simulink model "pedal_project"  (R2025b)
settings: Solver=VariableStepAuto  StartTime=0.0  StopTime=10.0  RelTol=1e-3
(part 1 of 2)

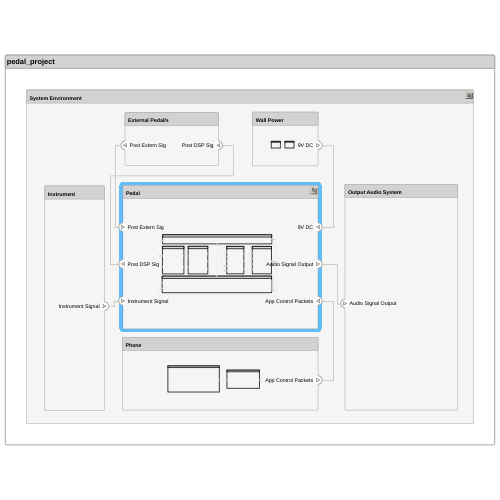
[thumbnail: Simulink's stored preview of the top-level diagram]
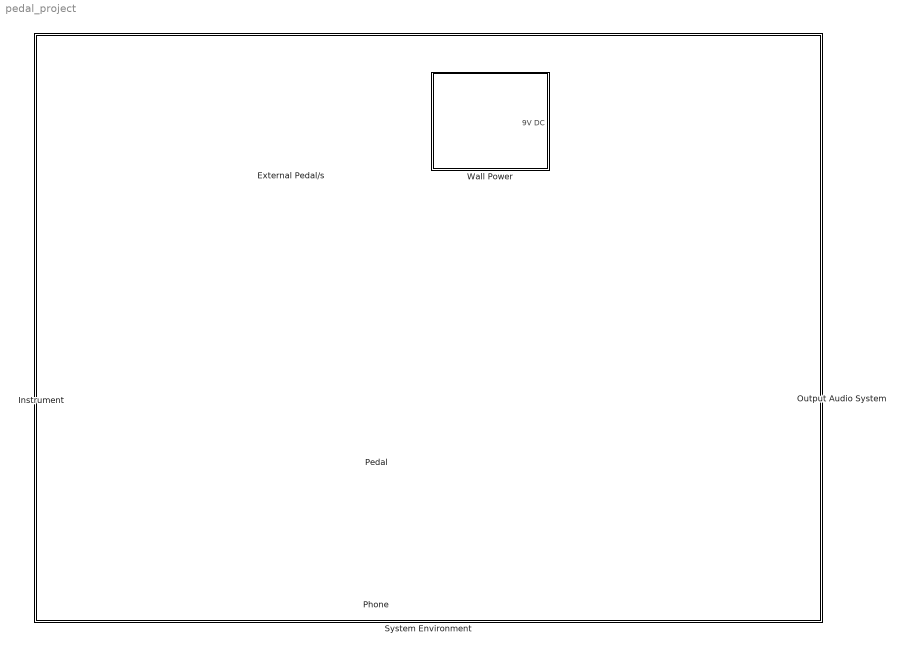
== system pedal_project ==
  External Pedal/s : Subsystem
      settings: PortSchema="{\"entries\":[{\"content\":{\"headerSize\":26,\"margin\":15,\"minimumSpacing\":25,\"sides\":[{\"content\":{\"connectorIds\":[\"Out1\"]},\"type\":\"ConnectorPlacement.EquallySpacedRectSide\",\"uuid\":\"d45e420a-c48a-4f64-96ce-c5c35bb4ca1a\"},{\"content\":{\"connectorIds\":[\"In1\"],\"side\":\"RIGHT\"},\"type\":\"ConnectorPlacement.EquallySpacedRectSide\",\"uuid\":\"a4e2bce0-d957-4e8d-907b-26e945724fec\"},{\"content\":{\"side\":\"TOP\"},\"type\":\"ConnectorPlacement.EquallySpacedRectSide\",\"uuid\":\"f887741f-84ea-4dc9-b916-61633ba77119\"},{\"content\":{\"side\":\"BOTTOM\"},\"type\":\"ConnectorPlacement.EquallySpacedRectSide\",\"uuid\":\"3b146cbf-c6c6-4afe-90ef-4dca6329af2e\"}]},\"type\":\"ConnectorPlacement.EquallySpacedConnector\",\"uuid\":\"ffda6ec7-3a8c-4734-85c7-d4d2baf408ab\"}],\"packageUris\":[\"http://schema.mathworks.com/mf0/Connector/R2020b\"],\"version\":\"1.0\"}"
  Instrument : Subsystem
      settings: PortSchema="{\"entries\":[{\"content\":{\"headerSize\":26,\"margin\":15,\"minimumSpacing\":25,\"sides\":[{\"content\":{},\"type\":\"ConnectorPlacement.EquallySpacedRectSide\",\"uuid\":\"d45e420a-c48a-4f64-96ce-c5c35bb4ca1a\"},{\"content\":{\"connectorIds\":[\"Out1\"],\"side\":\"RIGHT\"},\"type\":\"ConnectorPlacement.EquallySpacedRectSide\",\"uuid\":\"a4e2bce0-d957-4e8d-907b-26e945724fec\"},{\"content\":{\"side\":\"TOP\"},\"type\":\"ConnectorPlacement.EquallySpacedRectSide\",\"uuid\":\"f887741f-84ea-4dc9-b916-61633ba77119\"}]},\"type\":\"ConnectorPlacement.EquallySpacedConnector\",\"uuid\":\"ffda6ec7-3a8c-4734-85c7-d4d2baf408ab\"}],\"packageUris\":[\"http://schema.mathworks.com/mf0/Connector/R2020b\"],\"version\":\"1.0\"}"
  Output Audio System : Subsystem
      settings: PortSchema="{\"entries\":[{\"content\":{\"headerSize\":26,\"margin\":15,\"minimumSpacing\":25,\"sides\":[{\"content\":{\"connectorIds\":[\"In1\"]},\"type\":\"ConnectorPlacement.EquallySpacedRectSide\",\"uuid\":\"d45e420a-c48a-4f64-96ce-c5c35bb4ca1a\"},{\"content\":{\"side\":\"RIGHT\"},\"type\":\"ConnectorPlacement.EquallySpacedRectSide\",\"uuid\":\"a4e2bce0-d957-4e8d-907b-26e945724fec\"},{\"content\":{\"side\":\"TOP\"},\"type\":\"ConnectorPlacement.EquallySpacedRectSide\",\"uuid\":\"f887741f-84ea-4dc9-b916-61633ba77119\"}]},\"type\":\"ConnectorPlacement.EquallySpacedConnector\",\"uuid\":\"ffda6ec7-3a8c-4734-85c7-d4d2baf408ab\"}],\"packageUris\":[\"http://schema.mathworks.com/mf0/Connector/R2020b\"],\"version\":\"1.0\"}"
  Pedal : Subsystem
      settings: PortSchema="{\"entries\":[{\"content\":{\"headerSize\":26,\"margin\":15,\"minimumSpacing\":25,\"sides\":[{\"content\":{\"connectorIds\":[\"In3\",\"Out2\",\"In4\"]},\"type\":\"ConnectorPlacement.EquallySpacedRectSide\",\"uuid\":\"d45e420a-c48a-4f64-96ce-c5c35bb4ca1a\"},{\"content\":{\"connectorIds\":[\"In1\",\"Out1\",\"In2\"],\"side\":\"RIGHT\"},\"type\":\"ConnectorPlacement.EquallySpacedRectSide\",\"uuid\":\"a4e2bce0-d957-4e8d-907b-26e945724fec\"},{\"content\":{\"side\":\"TOP\"},\"type\":\"ConnectorPlacement.EquallySpacedRectSide\",\"uuid\":\"f887741f-84ea-4dc9-b916-61633ba77119\"}]},\"type\":\"ConnectorPlacement.EquallySpacedConnector\",\"uuid\":\"ffda6ec7-3a8c-4734-85c7-d4d2baf408ab\"}],\"packageUris\":[\"http://schema.mathworks.com/mf0/Connector/R2020b\"],\"version\":\"1.0\"}"
  Phone : Subsystem
      settings: PortSchema="{\"entries\":[{\"content\":{\"headerSize\":26,\"margin\":15,\"minimumSpacing\":25,\"sides\":[{\"content\":{},\"type\":\"ConnectorPlacement.EquallySpacedRectSide\",\"uuid\":\"d45e420a-c48a-4f64-96ce-c5c35bb4ca1a\"},{\"content\":{\"connectorIds\":[\"Out1\"],\"side\":\"RIGHT\"},\"type\":\"ConnectorPlacement.EquallySpacedRectSide\",\"uuid\":\"a4e2bce0-d957-4e8d-907b-26e945724fec\"},{\"content\":{\"side\":\"TOP\"},\"type\":\"ConnectorPlacement.EquallySpacedRectSide\",\"uuid\":\"f887741f-84ea-4dc9-b916-61633ba77119\"}]},\"type\":\"ConnectorPlacement.EquallySpacedConnector\",\"uuid\":\"ffda6ec7-3a8c-4734-85c7-d4d2baf408ab\"}],\"packageUris\":[\"http://schema.mathworks.com/mf0/Connector/R2020b\"],\"version\":\"1.0\"}"
  System Environment : Subsystem
      settings: PortSchema="{\"entries\":[{\"content\":{\"headerSize\":26,\"margin\":15,\"minimumSpacing\":25,\"sides\":[{\"content\":{},\"type\":\"ConnectorPlacement.EquallySpacedRectSide\",\"uuid\":\"ff6d08b7-25e5-4e55-8f49-6be1cf87a249\"},{\"content\":{\"side\":\"RIGHT\"},\"type\":\"ConnectorPlacement.EquallySpacedRectSide\",\"uuid\":\"cf714437-3edf-4193-96f0-527040f4845b\"},{\"content\":{\"side\":\"TOP\"},\"type\":\"ConnectorPlacement.EquallySpacedRectSide\",\"uuid\":\"edc7f9df-45d2-49f5-b248-99123dbc3df5\"}]},\"type\":\"ConnectorPlacement.EquallySpacedConnector\",\"uuid\":\"82090768-c12d-4d7c-bb71-6334bd2f3885\"}],\"packageUris\":[\"http://schema.mathworks.com/mf0/Connector/R2020b\"],\"version\":\"1.0\"}"
  Wall Power : Subsystem
      settings: PortSchema="{\"entries\":[{\"content\":{\"headerSize\":26,\"margin\":15,\"minimumSpacing\":25,\"sides\":[{\"content\":{},\"type\":\"ConnectorPlacement.EquallySpacedRectSide\",\"uuid\":\"d45e420a-c48a-4f64-96ce-c5c35bb4ca1a\"},{\"content\":{\"connectorIds\":[\"Out1\"],\"side\":\"RIGHT\"},\"type\":\"ConnectorPlacement.EquallySpacedRectSide\",\"uuid\":\"a4e2bce0-d957-4e8d-907b-26e945724fec\"},{\"content\":{\"side\":\"TOP\"},\"type\":\"ConnectorPlacement.EquallySpacedRectSide\",\"uuid\":\"f887741f-84ea-4dc9-b916-61633ba77119\"},{\"content\":{\"side\":\"BOTTOM\"},\"type\":\"ConnectorPlacement.EquallySpacedRectSide\",\"uuid\":\"d7988f96-c3a6-4963-bdc5-536baf489e90\"}]},\"type\":\"ConnectorPlacement.EquallySpacedConnector\",\"uuid\":\"ffda6ec7-3a8c-4734-85c7-d4d2baf408ab\"}],\"packageUris\":[\"http://schema.mathworks.com/mf0/Connector/R2020b\"],\"version\":\"1.0\"}"
  wires:
  Instrument/1(Instrument Signal) -> Pedal/4(Instrument Signal)
  Pedal/2(Post DSP Sig) -> External Pedal/s/1(Post DSP Sig)
  External Pedal/s/1(Post Extern Sig) -> Pedal/3(Post Extern Sig)
  Wall Power/1(9V DC) -> Pedal/1(9V DC)
  Phone/1(App Control Packets) -> Pedal/2(App Control Packets)
  Pedal/1(Audio Signal Output) -> Output Audio System/1(Audio Signal Output)

== system pedal_project/External Pedal//s ==
  Bus Element In1 : Inport  PortName=Post DSP Sig
  Bus Element Out1 : Outport  PortName=Post Extern Sig

== system pedal_project/Instrument ==
  Bus Element Out1 : Outport  PortName=Instrument Signal

== system pedal_project/Output Audio System ==
  Bus Element In1 : Inport  PortName=Audio Signal Output

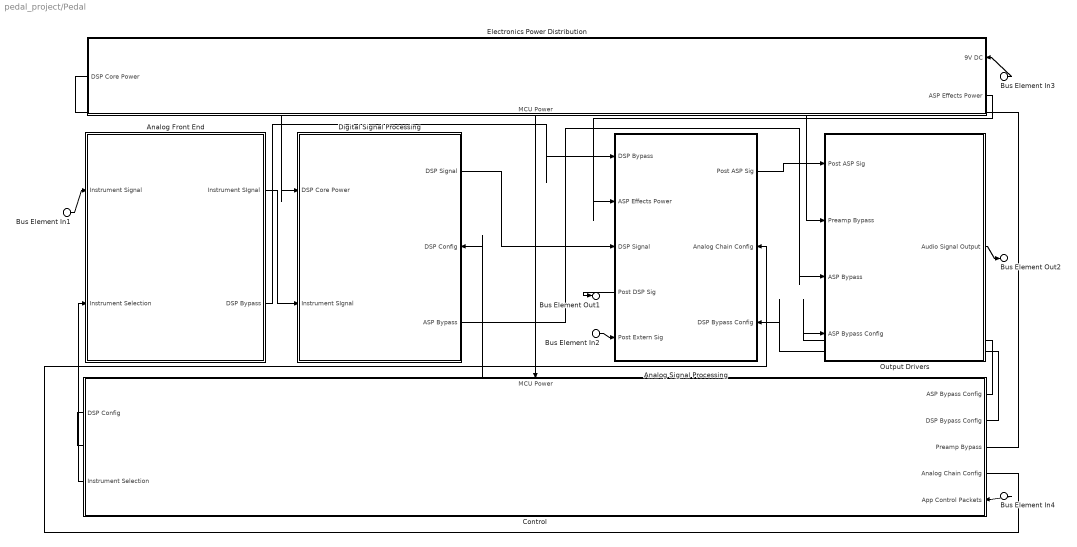
== system pedal_project/Pedal ==
  Bus Element In3 : Inport  PortName=9V DC
  Bus Element In4 : Inport  Port=2  PortName=App Control Packets
  Bus Element In2 : Inport  Port=3  PortName=Post Extern Sig
  Bus Element In1 : Inport  Port=4  PortName=Instrument Signal
  Analog Front End : Subsystem
      settings: PortSchema="{\"entries\":[{\"content\":{\"headerSize\":26,\"margin\":15,\"minimumSpacing\":25,\"sides\":[{\"content\":{\"connectorIds\":[\"In1\",\"In2\"]},\"type\":\"ConnectorPlacement.EquallySpacedRectSide\",\"uuid\":\"d45e420a-c48a-4f64-96ce-c5c35bb4ca1a\"},{\"content\":{\"connectorIds\":[\"Out1\",\"Out2\"],\"side\":\"RIGHT\"},\"type\":\"ConnectorPlacement.EquallySpacedRectSide\",\"uuid\":\"a4e2bce0-d957-4e8d-907b-26e945724fec\"},{\"content\":{\"side\":\"TOP\"},\"type\":\"ConnectorPlacement.EquallySpacedRectSide\",\"uuid\":\"f887741f-84ea-4dc9-b916-61633ba77119\"}]},\"type\":\"ConnectorPlacement.EquallySpacedConnector\",\"uuid\":\"ffda6ec7-3a8c-4734-85c7-d4d2baf408ab\"}],\"packageUris\":[\"http://schema.mathworks.com/mf0/Connector/R2020b\"],\"version\":\"1.0\"}"
  Analog Signal Processing : Subsystem
      settings: PortSchema="{\"entries\":[{\"content\":{\"headerSize\":26,\"margin\":15,\"minimumSpacing\":25,\"sides\":[{\"content\":{\"connectorIds\":[\"In1\",\"In3\",\"In4\",\"Out1\",\"In6\"]},\"type\":\"ConnectorPlacement.EquallySpacedRectSide\",\"uuid\":\"d45e420a-c48a-4f64-96ce-c5c35bb4ca1a\"},{\"content\":{\"connectorIds\":[\"Out2\",\"In5\",\"In2\"],\"side\":\"RIGHT\"},\"type\":\"ConnectorPlacement.EquallySpacedRectSide\",\"uuid\":\"a4e2bce0-d957-4e8d-907b-26e945724fec\"},{\"content\":{\"side\":\"TOP\"},\"type\":\"ConnectorPlacement.EquallySpacedRectSide\",\"uuid\":\"f887741f-84ea-4dc9-b916-61633ba77119\"}]},\"type\":\"ConnectorPlacement.EquallySpacedConnector\",\"uuid\":\"ffda6ec7-3a8c-4734-85c7-d4d2baf408ab\"}],\"packageUris\":[\"http://schema.mathworks.com/mf0/Connector/R2020b\"],\"version\":\"1.0\"}"
  Control : Subsystem
      settings: PortSchema="{\"entries\":[{\"content\":{\"headerSize\":26,\"margin\":15,\"minimumSpacing\":25,\"sides\":[{\"content\":{\"connectorIds\":[\"Out4\",\"Out5\"]},\"type\":\"ConnectorPlacement.EquallySpacedRectSide\",\"uuid\":\"d45e420a-c48a-4f64-96ce-c5c35bb4ca1a\"},{\"content\":{\"connectorIds\":[\"Out1\",\"Out2\",\"Out3\",\"Out6\",\"In1\"],\"side\":\"RIGHT\"},\"type\":\"ConnectorPlacement.EquallySpacedRectSide\",\"uuid\":\"a4e2bce0-d957-4e8d-907b-26e945724fec\"},{\"content\":{\"connectorIds\":[\"In2\"],\"side\":\"TOP\"},\"type\":\"ConnectorPlacement.EquallySpacedRectSide\",\"uuid\":\"f887741f-84ea-4dc9-b916-61633ba77119\"}]},\"type\":\"ConnectorPlacement.EquallySpacedConnector\",\"uuid\":\"ffda6ec7-3a8c-4734-85c7-d4d2baf408ab\"}],\"packageUris\":[\"http://schema.mathworks.com/mf0/Connector/R2020b\"],\"version\":\"1.0\"}"
  Digital Signal Processing : Subsystem
      settings: PortSchema="{\"entries\":[{\"content\":{\"headerSize\":26,\"margin\":15,\"minimumSpacing\":25,\"sides\":[{\"content\":{\"connectorIds\":[\"In1\",\"In3\"]},\"type\":\"ConnectorPlacement.EquallySpacedRectSide\",\"uuid\":\"d45e420a-c48a-4f64-96ce-c5c35bb4ca1a\"},{\"content\":{\"connectorIds\":[\"Out1\",\"In2\",\"Out2\"],\"side\":\"RIGHT\"},\"type\":\"ConnectorPlacement.EquallySpacedRectSide\",\"uuid\":\"a4e2bce0-d957-4e8d-907b-26e945724fec\"},{\"content\":{\"side\":\"TOP\"},\"type\":\"ConnectorPlacement.EquallySpacedRectSide\",\"uuid\":\"f887741f-84ea-4dc9-b916-61633ba77119\"}]},\"type\":\"ConnectorPlacement.EquallySpacedConnector\",\"uuid\":\"ffda6ec7-3a8c-4734-85c7-d4d2baf408ab\"}],\"packageUris\":[\"http://schema.mathworks.com/mf0/Connector/R2020b\"],\"version\":\"1.0\"}"
  Electronics Power Distribution : Subsystem
      settings: PortSchema="{\"entries\":[{\"content\":{\"headerSize\":26,\"margin\":15,\"minimumSpacing\":25,\"sides\":[{\"content\":{\"connectorIds\":[\"Out2\"]},\"type\":\"ConnectorPlacement.EquallySpacedRectSide\",\"uuid\":\"d45e420a-c48a-4f64-96ce-c5c35bb4ca1a\"},{\"content\":{\"connectorIds\":[\"In1\",\"Out1\"],\"side\":\"RIGHT\"},\"type\":\"ConnectorPlacement.EquallySpacedRectSide\",\"uuid\":\"a4e2bce0-d957-4e8d-907b-26e945724fec\"},{\"content\":{\"side\":\"TOP\"},\"type\":\"ConnectorPlacement.EquallySpacedRectSide\",\"uuid\":\"f887741f-84ea-4dc9-b916-61633ba77119\"},{\"content\":{\"connectorIds\":[\"Out3\"],\"side\":\"BOTTOM\"},\"type\":\"ConnectorPlacement.EquallySpacedRectSide\",\"uuid\":\"c9173022-6e53-493b-a07b-56b093cd8358\"}]},\"type\":\"ConnectorPlacement.EquallySpacedConnector\",\"uuid\":\"ffda6ec7-3a8c-4734-85c7-d4d2baf408ab\"}],\"packageUris\":[\"http://schema.mathworks.com/mf0/Connector/R2020b\"],\"version\":\"1.0\"}"
  Output Drivers : Subsystem
      settings: PortSchema="{\"entries\":[{\"content\":{\"headerSize\":26,\"margin\":15,\"minimumSpacing\":25,\"sides\":[{\"content\":{\"connectorIds\":[\"In1\",\"In2\",\"In3\",\"In4\"]},\"type\":\"ConnectorPlacement.EquallySpacedRectSide\",\"uuid\":\"d45e420a-c48a-4f64-96ce-c5c35bb4ca1a\"},{\"content\":{\"connectorIds\":[\"Out1\"],\"side\":\"RIGHT\"},\"type\":\"ConnectorPlacement.EquallySpacedRectSide\",\"uuid\":\"a4e2bce0-d957-4e8d-907b-26e945724fec\"},{\"content\":{\"side\":\"TOP\"},\"type\":\"ConnectorPlacement.EquallySpacedRectSide\",\"uuid\":\"f887741f-84ea-4dc9-b916-61633ba77119\"}]},\"type\":\"ConnectorPlacement.EquallySpacedConnector\",\"uuid\":\"ffda6ec7-3a8c-4734-85c7-d4d2baf408ab\"}],\"packageUris\":[\"http://schema.mathworks.com/mf0/Connector/R2020b\"],\"version\":\"1.0\"}"
  Bus Element Out2 : Outport  PortName=Audio Signal Output
  Bus Element Out1 : Outport  Port=2  PortName=Post DSP Sig
  wires:
  Electronics Power Distribution/3(MCU Power) -> Control/2(MCU Power)
  Bus Element In4/1 -> Control/1(App Control Packets)
  Output Drivers/1(Audio Signal Output) -> Bus Element Out2/1
  Bus Element In3/1 -> Electronics Power Distribution/1(9V DC)
  Bus Element In2/1 -> Analog Signal Processing/6(Post Extern Sig)
  Bus Element In1/1 -> Analog Front End/1(Instrument Signal)
  Analog Front End/1(Instrument SIgnal) -> Digital Signal Processing/3(Instrument SIgnal)
  Analog Signal Processing/2(Post ASP Sig) -> Output Drivers/1(Post ASP Sig)
  Control/6(Analog Chain Config) -> Analog Signal Processing/5(Analog Chain Config)
  Control/4(DSP Config) -> Digital Signal Processing/2(DSP Config)
  Control/5(Instrument Selection) -> Analog Front End/2(Instrument Selection)
  Electronics Power Distribution/2(DSP Core Power) -> Digital Signal Processing/1(DSP Core Power)
  Electronics Power Distribution/1(ASP Effects Power) -> Analog Signal Processing/3(ASP Effects Power)
  Analog Signal Processing/1(Post DSP Sig) -> Bus Element Out1/1
  Digital Signal Processing/1(DSP Signal) -> Analog Signal Processing/4(DSP Signal)
  Control/3(Preamp Bypass) -> Output Drivers/2(Preamp Bypass)
  Digital Signal Processing/2(ASP Bypass) -> Output Drivers/3(ASP Bypass)
  Analog Front End/2(DSP Bypass) -> Analog Signal Processing/1(DSP Bypass)
  Control/2(DSP Bypass Config) -> Analog Signal Processing/2(DSP Bypass Config)
  Control/1(ASP Bypass Config) -> Output Drivers/4(ASP Bypass Config)

== system pedal_project/Phone ==
  Software Application : Subsystem
      settings: PortSchema="{\"entries\":[{\"content\":{\"headerSize\":26,\"margin\":15,\"minimumSpacing\":25,\"sides\":[{\"content\":{},\"type\":\"ConnectorPlacement.EquallySpacedRectSide\",\"uuid\":\"d45e420a-c48a-4f64-96ce-c5c35bb4ca1a\"},{\"content\":{\"connectorIds\":[\"Out1\"],\"side\":\"RIGHT\"},\"type\":\"ConnectorPlacement.EquallySpacedRectSide\",\"uuid\":\"a4e2bce0-d957-4e8d-907b-26e945724fec\"},{\"content\":{\"side\":\"TOP\"},\"type\":\"ConnectorPlacement.EquallySpacedRectSide\",\"uuid\":\"f887741f-84ea-4dc9-b916-61633ba77119\"}]},\"type\":\"ConnectorPlacement.EquallySpacedConnector\",\"uuid\":\"ffda6ec7-3a8c-4734-85c7-d4d2baf408ab\"}],\"packageUris\":[\"http://schema.mathworks.com/mf0/Connector/R2020b\"],\"version\":\"1.0\"}"
  USB Output Driver : Subsystem
      settings: PortSchema="{\"entries\":[{\"content\":{\"headerSize\":26,\"margin\":15,\"minimumSpacing\":25,\"sides\":[{\"content\":{\"connectorIds\":[\"In1\"]},\"type\":\"ConnectorPlacement.EquallySpacedRectSide\",\"uuid\":\"d45e420a-c48a-4f64-96ce-c5c35bb4ca1a\"},{\"content\":{\"connectorIds\":[\"Out1\"],\"side\":\"RIGHT\"},\"type\":\"ConnectorPlacement.EquallySpacedRectSide\",\"uuid\":\"a4e2bce0-d957-4e8d-907b-26e945724fec\"},{\"content\":{\"side\":\"TOP\"},\"type\":\"ConnectorPlacement.EquallySpacedRectSide\",\"uuid\":\"f887741f-84ea-4dc9-b916-61633ba77119\"}]},\"type\":\"ConnectorPlacement.EquallySpacedConnector\",\"uuid\":\"ffda6ec7-3a8c-4734-85c7-d4d2baf408ab\"}],\"packageUris\":[\"http://schema.mathworks.com/mf0/Connector/R2020b\"],\"version\":\"1.0\"}"
  Bus Element Out1 : Outport  PortName=App Control Packets
  wires:
  USB Output Driver/1(App Control Packets) -> Bus Element Out1/1
  Software Application/1(Configuration Upload Packets) -> USB Output Driver/1(Configuration Upload Packets)

== system pedal_project/System Environment ==

== system pedal_project/Wall Power ==
  120V Wall Output : Subsystem
      settings: PortSchema="{\"entries\":[{\"content\":{\"headerSize\":26,\"margin\":15,\"minimumSpacing\":25,\"sides\":[{\"content\":{},\"type\":\"ConnectorPlacement.EquallySpacedRectSide\",\"uuid\":\"d45e420a-c48a-4f64-96ce-c5c35bb4ca1a\"},{\"content\":{\"connectorIds\":[\"Out1\"],\"side\":\"RIGHT\"},\"type\":\"ConnectorPlacement.EquallySpacedRectSide\",\"uuid\":\"a4e2bce0-d957-4e8d-907b-26e945724fec\"},{\"content\":{\"side\":\"TOP\"},\"type\":\"ConnectorPlacement.EquallySpacedRectSide\",\"uuid\":\"f887741f-84ea-4dc9-b916-61633ba77119\"}]},\"type\":\"ConnectorPlacement.EquallySpacedConnector\",\"uuid\":\"ffda6ec7-3a8c-4734-85c7-d4d2baf408ab\"}],\"packageUris\":[\"http://schema.mathworks.com/mf0/Connector/R2020b\"],\"version\":\"1.0\"}"
  9V DC Power Supply : Subsystem
      settings: PortSchema="{\"entries\":[{\"content\":{\"headerSize\":26,\"margin\":15,\"minimumSpacing\":25,\"sides\":[{\"content\":{\"connectorIds\":[\"In1\"]},\"type\":\"ConnectorPlacement.EquallySpacedRectSide\",\"uuid\":\"d45e420a-c48a-4f64-96ce-c5c35bb4ca1a\"},{\"content\":{\"connectorIds\":[\"Out1\"],\"side\":\"RIGHT\"},\"type\":\"ConnectorPlacement.EquallySpacedRectSide\",\"uuid\":\"a4e2bce0-d957-4e8d-907b-26e945724fec\"},{\"content\":{\"side\":\"TOP\"},\"type\":\"ConnectorPlacement.EquallySpacedRectSide\",\"uuid\":\"f887741f-84ea-4dc9-b916-61633ba77119\"}]},\"type\":\"ConnectorPlacement.EquallySpacedConnector\",\"uuid\":\"ffda6ec7-3a8c-4734-85c7-d4d2baf408ab\"}],\"packageUris\":[\"http://schema.mathworks.com/mf0/Connector/R2020b\"],\"version\":\"1.0\"}"
  Bus Element Out1 : Outport  PortName=9V DC
  wires:
  120V Wall Output/1(Wall Power) -> 9V DC Power Supply/1(Wall Power)
  9V DC Power Supply/1(9V DC) -> Bus Element Out1/1

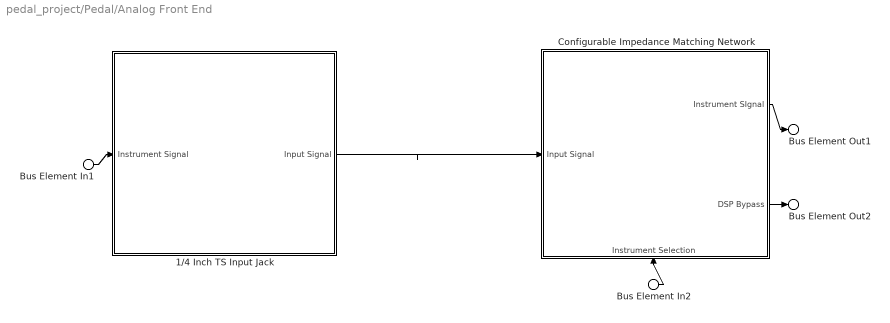
== system pedal_project/Pedal/Analog Front End ==
  Bus Element In1 : Inport  PortName=Instrument Signal
  Bus Element In2 : Inport  Port=2  PortName=Instrument Selection
  1/4 Inch TS Input Jack : Subsystem
      settings: PortSchema="{\"entries\":[{\"content\":{\"headerSize\":26,\"margin\":15,\"minimumSpacing\":25,\"sides\":[{\"content\":{\"connectorIds\":[\"In1\"]},\"type\":\"ConnectorPlacement.EquallySpacedRectSide\",\"uuid\":\"d45e420a-c48a-4f64-96ce-c5c35bb4ca1a\"},{\"content\":{\"connectorIds\":[\"Out1\"],\"side\":\"RIGHT\"},\"type\":\"ConnectorPlacement.EquallySpacedRectSide\",\"uuid\":\"a4e2bce0-d957-4e8d-907b-26e945724fec\"},{\"content\":{\"side\":\"TOP\"},\"type\":\"ConnectorPlacement.EquallySpacedRectSide\",\"uuid\":\"f887741f-84ea-4dc9-b916-61633ba77119\"}]},\"type\":\"ConnectorPlacement.EquallySpacedConnector\",\"uuid\":\"ffda6ec7-3a8c-4734-85c7-d4d2baf408ab\"}],\"packageUris\":[\"http://schema.mathworks.com/mf0/Connector/R2020b\"],\"version\":\"1.0\"}"
  Configurable Impedance Matching Network : Subsystem
      settings: PortSchema="{\"entries\":[{\"content\":{\"headerSize\":26,\"margin\":15,\"minimumSpacing\":25,\"sides\":[{\"content\":{\"connectorIds\":[\"In2\"]},\"type\":\"ConnectorPlacement.EquallySpacedRectSide\",\"uuid\":\"d45e420a-c48a-4f64-96ce-c5c35bb4ca1a\"},{\"content\":{\"connectorIds\":[\"Out1\",\"Out2\"],\"side\":\"RIGHT\"},\"type\":\"ConnectorPlacement.EquallySpacedRectSide\",\"uuid\":\"a4e2bce0-d957-4e8d-907b-26e945724fec\"},{\"content\":{\"side\":\"TOP\"},\"type\":\"ConnectorPlacement.EquallySpacedRectSide\",\"uuid\":\"f887741f-84ea-4dc9-b916-61633ba77119\"},{\"content\":{\"connectorIds\":[\"In1\"],\"side\":\"BOTTOM\"},\"type\":\"ConnectorPlacement.EquallySpacedRectSide\",\"uuid\":\"a508731f-4cdb-4416-a773-6d2230bc93f7\"}]},\"type\":\"ConnectorPlacement.EquallySpacedConnector\",\"uuid\":\"ffda6ec7-3a8c-4734-85c7-d4d2baf408ab\"}],\"packageUris\":[\"http://schema.mathworks.com/mf0/Connector/R2020b\"],\"version\":\"1.0\"}"
  Bus Element Out1 : Outport  PortName=Instrument SIgnal
  Bus Element Out2 : Outport  Port=2  PortName=DSP Bypass
  wires:
  Bus Element In1/1 -> 1/4 Inch TS Input Jack/1(Instrument Signal)
  1/4 Inch TS Input Jack/1(Input Signal) -> Configurable Impedance Matching Network/2(Input Signal)
  Configurable Impedance Matching Network/1(Instrument SIgnal) -> Bus Element Out1/1
  Bus Element In2/1 -> Configurable Impedance Matching Network/1(Instrument Selection)
  Configurable Impedance Matching Network/2(DSP Bypass) -> Bus Element Out2/1

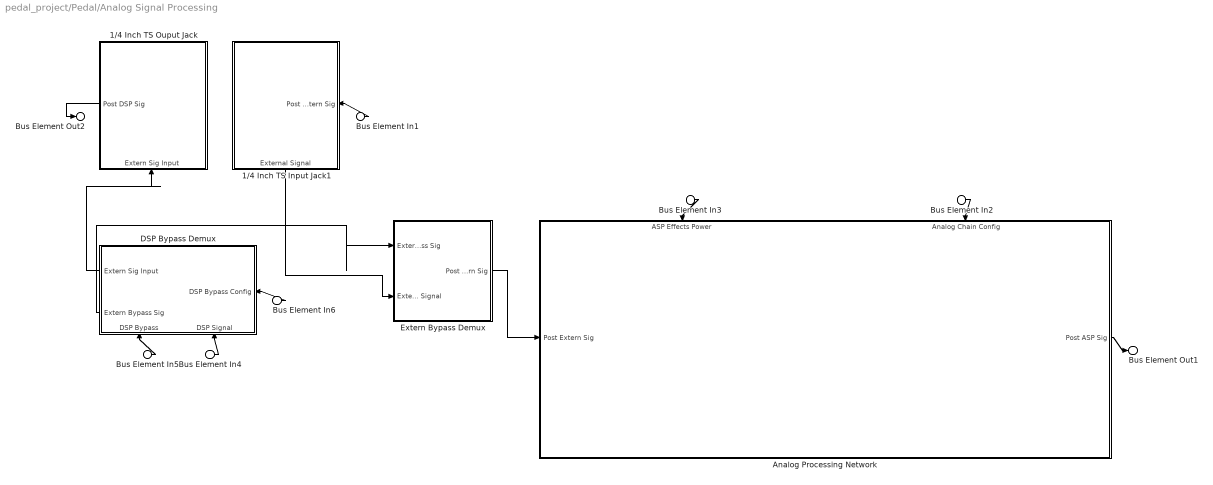
== system pedal_project/Pedal/Analog Signal Processing ==
  Bus Element In5 : Inport  PortName=DSP Bypass
  Bus Element In6 : Inport  Port=2  PortName=DSP Bypass Config
  Bus Element In3 : Inport  Port=3  PortName=ASP Effects Power
  Bus Element In4 : Inport  Port=4  PortName=DSP Signal
  Bus Element In2 : Inport  Port=5  PortName=Analog Chain Config
  Bus Element In1 : Inport  Port=6  PortName=Post Extern Sig
  1/4 Inch TS Input Jack1 : Subsystem
      settings: PortSchema="{\"entries\":[{\"content\":{\"headerSize\":26,\"margin\":15,\"minimumSpacing\":25,\"sides\":[{\"content\":{},\"type\":\"ConnectorPlacement.EquallySpacedRectSide\",\"uuid\":\"d45e420a-c48a-4f64-96ce-c5c35bb4ca1a\"},{\"content\":{\"connectorIds\":[\"In1\"],\"side\":\"RIGHT\"},\"type\":\"ConnectorPlacement.EquallySpacedRectSide\",\"uuid\":\"a4e2bce0-d957-4e8d-907b-26e945724fec\"},{\"content\":{\"side\":\"TOP\"},\"type\":\"ConnectorPlacement.EquallySpacedRectSide\",\"uuid\":\"f887741f-84ea-4dc9-b916-61633ba77119\"},{\"content\":{\"connectorIds\":[\"Out1\"],\"side\":\"BOTTOM\"},\"type\":\"ConnectorPlacement.EquallySpacedRectSide\",\"uuid\":\"a2e99f68-b657-45db-b83d-83257bff40de\"}]},\"type\":\"ConnectorPlacement.EquallySpacedConnector\",\"uuid\":\"ffda6ec7-3a8c-4734-85c7-d4d2baf408ab\"}],\"packageUris\":[\"http://schema.mathworks.com/mf0/Connector/R2020b\"],\"version\":\"1.0\"}"
  1/4 Inch TS Ouput Jack : Subsystem
      settings: PortSchema="{\"entries\":[{\"content\":{\"headerSize\":26,\"margin\":15,\"minimumSpacing\":25,\"sides\":[{\"content\":{\"connectorIds\":[\"Out1\"]},\"type\":\"ConnectorPlacement.EquallySpacedRectSide\",\"uuid\":\"d45e420a-c48a-4f64-96ce-c5c35bb4ca1a\"},{\"content\":{\"side\":\"RIGHT\"},\"type\":\"ConnectorPlacement.EquallySpacedRectSide\",\"uuid\":\"a4e2bce0-d957-4e8d-907b-26e945724fec\"},{\"content\":{\"side\":\"TOP\"},\"type\":\"ConnectorPlacement.EquallySpacedRectSide\",\"uuid\":\"f887741f-84ea-4dc9-b916-61633ba77119\"},{\"content\":{\"connectorIds\":[\"In1\"],\"side\":\"BOTTOM\"},\"type\":\"ConnectorPlacement.EquallySpacedRectSide\",\"uuid\":\"88965f48-d143-40f6-91a4-d37ed6aa82cc\"}]},\"type\":\"ConnectorPlacement.EquallySpacedConnector\",\"uuid\":\"ffda6ec7-3a8c-4734-85c7-d4d2baf408ab\"}],\"packageUris\":[\"http://schema.mathworks.com/mf0/Connector/R2020b\"],\"version\":\"1.0\"}"
  Analog Processing Network : Subsystem
      settings: PortSchema="{\"entries\":[{\"content\":{\"headerSize\":26,\"margin\":15,\"minimumSpacing\":25,\"sides\":[{\"content\":{\"connectorIds\":[\"In1\"]},\"type\":\"ConnectorPlacement.EquallySpacedRectSide\",\"uuid\":\"d45e420a-c48a-4f64-96ce-c5c35bb4ca1a\"},{\"content\":{\"connectorIds\":[\"Out1\"],\"side\":\"RIGHT\"},\"type\":\"ConnectorPlacement.EquallySpacedRectSide\",\"uuid\":\"a4e2bce0-d957-4e8d-907b-26e945724fec\"},{\"content\":{\"connectorIds\":[\"In2\",\"In3\"],\"side\":\"TOP\"},\"type\":\"ConnectorPlacement.EquallySpacedRectSide\",\"uuid\":\"f887741f-84ea-4dc9-b916-61633ba77119\"}]},\"type\":\"ConnectorPlacement.EquallySpacedConnector\",\"uuid\":\"ffda6ec7-3a8c-4734-85c7-d4d2baf408ab\"}],\"packageUris\":[\"http://schema.mathworks.com/mf0/Connector/R2020b\"],\"version\":\"1.0\"}"
  DSP Bypass Demux : Subsystem
      settings: PortSchema="{\"entries\":[{\"content\":{\"headerSize\":26,\"margin\":15,\"minimumSpacing\":25,\"sides\":[{\"content\":{\"connectorIds\":[\"Out1\",\"Out2\"]},\"type\":\"ConnectorPlacement.EquallySpacedRectSide\",\"uuid\":\"d45e420a-c48a-4f64-96ce-c5c35bb4ca1a\"},{\"content\":{\"connectorIds\":[\"In1\"],\"side\":\"RIGHT\"},\"type\":\"ConnectorPlacement.EquallySpacedRectSide\",\"uuid\":\"a4e2bce0-d957-4e8d-907b-26e945724fec\"},{\"content\":{\"side\":\"TOP\"},\"type\":\"ConnectorPlacement.EquallySpacedRectSide\",\"uuid\":\"f887741f-84ea-4dc9-b916-61633ba77119\"},{\"content\":{\"connectorIds\":[\"In2\",\"In3\"],\"side\":\"BOTTOM\"},\"type\":\"ConnectorPlacement.EquallySpacedRectSide\",\"uuid\":\"a9cbd870-749e-4f72-9453-e2059894359a\"}]},\"type\":\"ConnectorPlacement.EquallySpacedConnector\",\"uuid\":\"ffda6ec7-3a8c-4734-85c7-d4d2baf408ab\"}],\"packageUris\":[\"http://schema.mathworks.com/mf0/Connector/R2020b\"],\"version\":\"1.0\"}"
  Extern Bypass Demux : Subsystem
      settings: PortSchema="{\"entries\":[{\"content\":{\"headerSize\":26,\"margin\":15,\"minimumSpacing\":25,\"sides\":[{\"content\":{\"connectorIds\":[\"In1\",\"In2\"]},\"type\":\"ConnectorPlacement.EquallySpacedRectSide\",\"uuid\":\"d45e420a-c48a-4f64-96ce-c5c35bb4ca1a\"},{\"content\":{\"connectorIds\":[\"Out1\"],\"side\":\"RIGHT\"},\"type\":\"ConnectorPlacement.EquallySpacedRectSide\",\"uuid\":\"a4e2bce0-d957-4e8d-907b-26e945724fec\"},{\"content\":{\"side\":\"TOP\"},\"type\":\"ConnectorPlacement.EquallySpacedRectSide\",\"uuid\":\"f887741f-84ea-4dc9-b916-61633ba77119\"}]},\"type\":\"ConnectorPlacement.EquallySpacedConnector\",\"uuid\":\"ffda6ec7-3a8c-4734-85c7-d4d2baf408ab\"}],\"packageUris\":[\"http://schema.mathworks.com/mf0/Connector/R2020b\"],\"version\":\"1.0\"}"
  Bus Element Out2 : Outport  PortName=Post DSP Sig
  Bus Element Out1 : Outport  Port=2  PortName=Post ASP Sig
  wires:
  1/4 Inch TS Ouput Jack/1(Post DSP Sig) -> Bus Element Out2/1
  Bus Element In1/1 -> 1/4 Inch TS Input Jack1/1(Post Extern Sig)
  Bus Element In3/1 -> Analog Processing Network/2(ASP Effects Power)
  Analog Processing Network/1(Post ASP Sig) -> Bus Element Out1/1
  Bus Element In2/1 -> Analog Processing Network/3(Analog Chain Config)
  Bus Element In4/1 -> DSP Bypass Demux/3(DSP Signal)
  Bus Element In5/1 -> DSP Bypass Demux/2(DSP Bypass)
  DSP Bypass Demux/1(Extern Sig Input) -> 1/4 Inch TS Ouput Jack/1(Extern Sig Input)
  Bus Element In6/1 -> DSP Bypass Demux/1(DSP Bypass Config)
  1/4 Inch TS Input Jack1/1(External Signal) -> Extern Bypass Demux/2(External Signal)
  DSP Bypass Demux/2(Extern Bypass Sig) -> Extern Bypass Demux/1(Extern Bypass Sig)
  Extern Bypass Demux/1(Post Extern Sig) -> Analog Processing Network/1(Post Extern Sig)

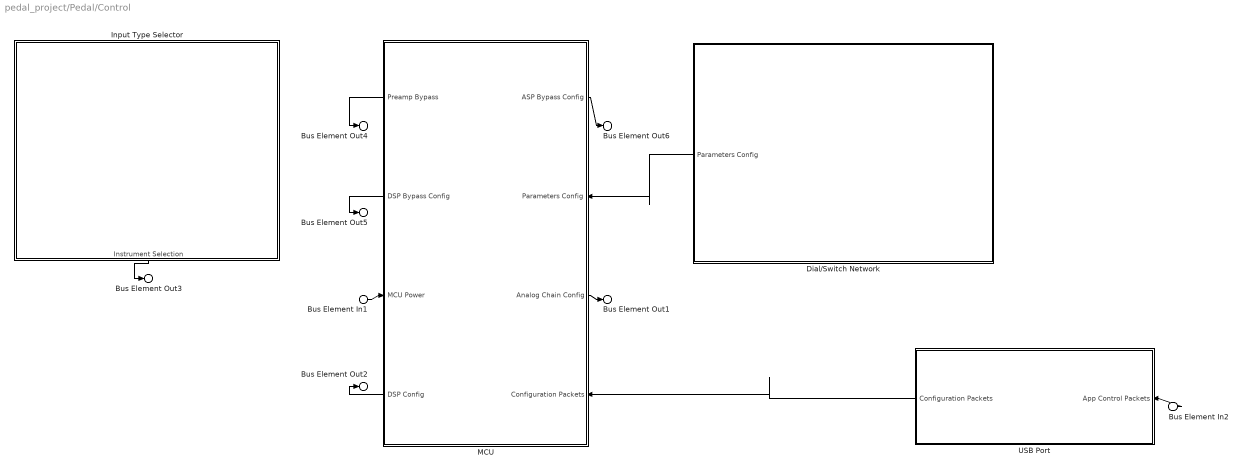
== system pedal_project/Pedal/Control ==
  Bus Element In2 : Inport  PortName=App Control Packets
  Bus Element In1 : Inport  Port=2  PortName=MCU Power
  Dial/Switch Network : Subsystem
      settings: PortSchema="{\"entries\":[{\"content\":{\"headerSize\":26,\"margin\":15,\"minimumSpacing\":25,\"sides\":[{\"content\":{\"connectorIds\":[\"Out1\"]},\"type\":\"ConnectorPlacement.EquallySpacedRectSide\",\"uuid\":\"d45e420a-c48a-4f64-96ce-c5c35bb4ca1a\"},{\"content\":{\"side\":\"RIGHT\"},\"type\":\"ConnectorPlacement.EquallySpacedRectSide\",\"uuid\":\"a4e2bce0-d957-4e8d-907b-26e945724fec\"},{\"content\":{\"side\":\"TOP\"},\"type\":\"ConnectorPlacement.EquallySpacedRectSide\",\"uuid\":\"f887741f-84ea-4dc9-b916-61633ba77119\"}]},\"type\":\"ConnectorPlacement.EquallySpacedConnector\",\"uuid\":\"ffda6ec7-3a8c-4734-85c7-d4d2baf408ab\"}],\"packageUris\":[\"http://schema.mathworks.com/mf0/Connector/R2020b\"],\"version\":\"1.0\"}"
  Input Type Selector : Subsystem
      settings: PortSchema="{\"entries\":[{\"content\":{\"headerSize\":26,\"margin\":15,\"minimumSpacing\":25,\"sides\":[{\"content\":{},\"type\":\"ConnectorPlacement.EquallySpacedRectSide\",\"uuid\":\"d45e420a-c48a-4f64-96ce-c5c35bb4ca1a\"},{\"content\":{\"side\":\"RIGHT\"},\"type\":\"ConnectorPlacement.EquallySpacedRectSide\",\"uuid\":\"a4e2bce0-d957-4e8d-907b-26e945724fec\"},{\"content\":{\"side\":\"TOP\"},\"type\":\"ConnectorPlacement.EquallySpacedRectSide\",\"uuid\":\"f887741f-84ea-4dc9-b916-61633ba77119\"},{\"content\":{\"connectorIds\":[\"Out1\"],\"side\":\"BOTTOM\"},\"type\":\"ConnectorPlacement.EquallySpacedRectSide\",\"uuid\":\"d54f53cd-426d-4f62-aea0-61e554017ffa\"}]},\"type\":\"ConnectorPlacement.EquallySpacedConnector\",\"uuid\":\"ffda6ec7-3a8c-4734-85c7-d4d2baf408ab\"}],\"packageUris\":[\"http://schema.mathworks.com/mf0/Connector/R2020b\"],\"version\":\"1.0\"}"
  MCU : Subsystem
      settings: PortSchema="{\"entries\":[{\"content\":{\"headerSize\":26,\"margin\":15,\"minimumSpacing\":25,\"sides\":[{\"content\":{\"connectorIds\":[\"Out2\",\"Out3\",\"In1\",\"Out5\"]},\"type\":\"ConnectorPlacement.EquallySpacedRectSide\",\"uuid\":\"d45e420a-c48a-4f64-96ce-c5c35bb4ca1a\"},{\"content\":{\"connectorIds\":[\"Out1\",\"In2\",\"Out4\",\"In3\"],\"side\":\"RIGHT\"},\"type\":\"ConnectorPlacement.EquallySpacedRectSide\",\"uuid\":\"a4e2bce0-d957-4e8d-907b-26e945724fec\"},{\"content\":{\"side\":\"TOP\"},\"type\":\"ConnectorPlacement.EquallySpacedRectSide\",\"uuid\":\"f887741f-84ea-4dc9-b916-61633ba77119\"}]},\"type\":\"ConnectorPlacement.EquallySpacedConnector\",\"uuid\":\"ffda6ec7-3a8c-4734-85c7-d4d2baf408ab\"}],\"packageUris\":[\"http://schema.mathworks.com/mf0/Connector/R2020b\"],\"version\":\"1.0\"}"
  USB Port : Subsystem
      settings: PortSchema="{\"entries\":[{\"content\":{\"headerSize\":26,\"margin\":15,\"minimumSpacing\":25,\"sides\":[{\"content\":{\"connectorIds\":[\"Out1\"]},\"type\":\"ConnectorPlacement.EquallySpacedRectSide\",\"uuid\":\"d45e420a-c48a-4f64-96ce-c5c35bb4ca1a\"},{\"content\":{\"connectorIds\":[\"In1\"],\"side\":\"RIGHT\"},\"type\":\"ConnectorPlacement.EquallySpacedRectSide\",\"uuid\":\"a4e2bce0-d957-4e8d-907b-26e945724fec\"},{\"content\":{\"side\":\"TOP\"},\"type\":\"ConnectorPlacement.EquallySpacedRectSide\",\"uuid\":\"f887741f-84ea-4dc9-b916-61633ba77119\"}]},\"type\":\"ConnectorPlacement.EquallySpacedConnector\",\"uuid\":\"ffda6ec7-3a8c-4734-85c7-d4d2baf408ab\"}],\"packageUris\":[\"http://schema.mathworks.com/mf0/Connector/R2020b\"],\"version\":\"1.0\"}"
  Bus Element Out6 : Outport  PortName=ASP Bypass Config
  Bus Element Out5 : Outport  Port=2  PortName=DSP Bypass Config
  Bus Element Out4 : Outport  Port=3  PortName=Preamp Bypass
  Bus Element Out2 : Outport  Port=4  PortName=DSP Config
  Bus Element Out3 : Outport  Port=5  PortName=Instrument Selection
  Bus Element Out1 : Outport  Port=6  PortName=Analog Chain Config
  wires:
  Bus Element In2/1 -> USB Port/1(App Control Packets)
  MCU/5(DSP Config) -> Bus Element Out2/1
  Input Type Selector/1(Instrument Selection) -> Bus Element Out3/1
  MCU/4(Analog Chain Config) -> Bus Element Out1/1
  Dial/Switch Network/1(Parameters Config) -> MCU/2(Parameters Config)
  USB Port/1(Configuration Packets) -> MCU/3(Configuration Packets)
  Bus Element In1/1 -> MCU/1(MCU Power)
  MCU/3(DSP Bypass Config) -> Bus Element Out5/1
  MCU/2(Preamp Bypass) -> Bus Element Out4/1
  MCU/1(ASP Bypass Config) -> Bus Element Out6/1

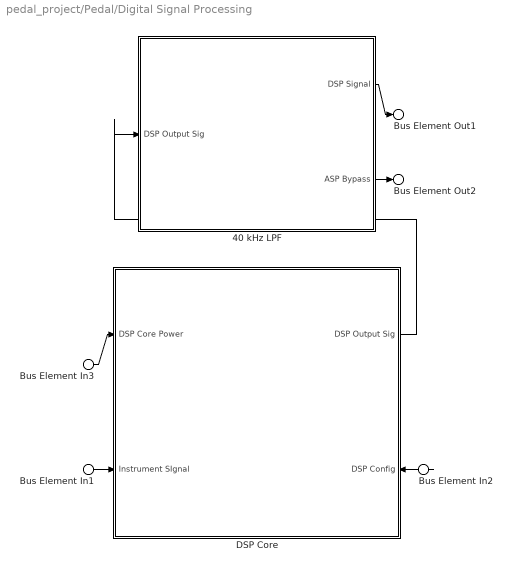
== system pedal_project/Pedal/Digital Signal Processing ==
  Bus Element In3 : Inport  PortName=DSP Core Power
  Bus Element In2 : Inport  Port=2  PortName=DSP Config
  Bus Element In1 : Inport  Port=3  PortName=Instrument SIgnal
  40 kHz LPF : Subsystem
      settings: PortSchema="{\"entries\":[{\"content\":{\"headerSize\":26,\"margin\":15,\"minimumSpacing\":25,\"sides\":[{\"content\":{\"connectorIds\":[\"In1\"]},\"type\":\"ConnectorPlacement.EquallySpacedRectSide\",\"uuid\":\"d45e420a-c48a-4f64-96ce-c5c35bb4ca1a\"},{\"content\":{\"connectorIds\":[\"Out1\",\"Out2\"],\"side\":\"RIGHT\"},\"type\":\"ConnectorPlacement.EquallySpacedRectSide\",\"uuid\":\"a4e2bce0-d957-4e8d-907b-26e945724fec\"},{\"content\":{\"side\":\"TOP\"},\"type\":\"ConnectorPlacement.EquallySpacedRectSide\",\"uuid\":\"f887741f-84ea-4dc9-b916-61633ba77119\"}]},\"type\":\"ConnectorPlacement.EquallySpacedConnector\",\"uuid\":\"ffda6ec7-3a8c-4734-85c7-d4d2baf408ab\"}],\"packageUris\":[\"http://schema.mathworks.com/mf0/Connector/R2020b\"],\"version\":\"1.0\"}"
  DSP Core : Subsystem
      settings: PortSchema="{\"entries\":[{\"content\":{\"headerSize\":26,\"margin\":15,\"minimumSpacing\":25,\"sides\":[{\"content\":{\"connectorIds\":[\"In2\",\"In3\"]},\"type\":\"ConnectorPlacement.EquallySpacedRectSide\",\"uuid\":\"d45e420a-c48a-4f64-96ce-c5c35bb4ca1a\"},{\"content\":{\"connectorIds\":[\"Out1\",\"In1\"],\"side\":\"RIGHT\"},\"type\":\"ConnectorPlacement.EquallySpacedRectSide\",\"uuid\":\"a4e2bce0-d957-4e8d-907b-26e945724fec\"},{\"content\":{\"side\":\"TOP\"},\"type\":\"ConnectorPlacement.EquallySpacedRectSide\",\"uuid\":\"f887741f-84ea-4dc9-b916-61633ba77119\"}]},\"type\":\"ConnectorPlacement.EquallySpacedConnector\",\"uuid\":\"ffda6ec7-3a8c-4734-85c7-d4d2baf408ab\"}],\"packageUris\":[\"http://schema.mathworks.com/mf0/Connector/R2020b\"],\"version\":\"1.0\"}"
  Bus Element Out1 : Outport  PortName=DSP Signal
  Bus Element Out2 : Outport  Port=2  PortName=ASP Bypass
  wires:
  Bus Element In1/1 -> DSP Core/3(Instrument SIgnal)
  Bus Element In3/1 -> DSP Core/2(DSP Core Power)
  Bus Element In2/1 -> DSP Core/1(DSP Config)
  DSP Core/1(DSP Output Sig) -> 40 kHz LPF/1(DSP Output Sig)
  40 kHz LPF/1(DSP Signal) -> Bus Element Out1/1
  40 kHz LPF/2(ASP Bypass) -> Bus Element Out2/1

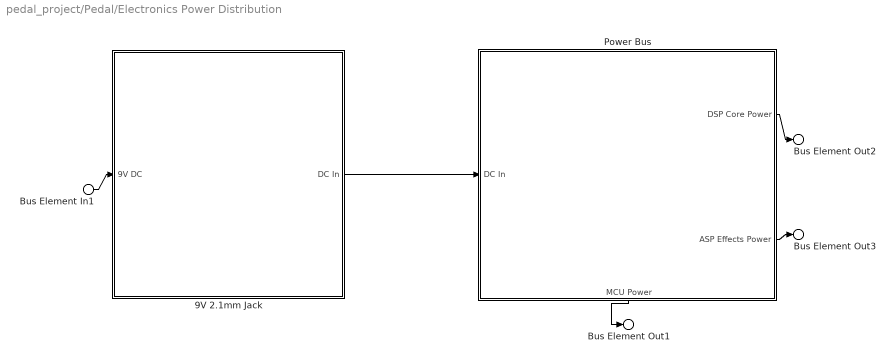
== system pedal_project/Pedal/Electronics Power Distribution ==
  Bus Element In1 : Inport  PortName=9V DC
  9V 2.1mm Jack : Subsystem
      settings: PortSchema="{\"entries\":[{\"content\":{\"headerSize\":26,\"margin\":15,\"minimumSpacing\":25,\"sides\":[{\"content\":{\"connectorIds\":[\"In1\"]},\"type\":\"ConnectorPlacement.EquallySpacedRectSide\",\"uuid\":\"d45e420a-c48a-4f64-96ce-c5c35bb4ca1a\"},{\"content\":{\"connectorIds\":[\"Out1\"],\"side\":\"RIGHT\"},\"type\":\"ConnectorPlacement.EquallySpacedRectSide\",\"uuid\":\"a4e2bce0-d957-4e8d-907b-26e945724fec\"},{\"content\":{\"side\":\"TOP\"},\"type\":\"ConnectorPlacement.EquallySpacedRectSide\",\"uuid\":\"f887741f-84ea-4dc9-b916-61633ba77119\"}]},\"type\":\"ConnectorPlacement.EquallySpacedConnector\",\"uuid\":\"ffda6ec7-3a8c-4734-85c7-d4d2baf408ab\"}],\"packageUris\":[\"http://schema.mathworks.com/mf0/Connector/R2020b\"],\"version\":\"1.0\"}"
  Power Bus : Subsystem
      settings: PortSchema="{\"entries\":[{\"content\":{\"headerSize\":26,\"margin\":15,\"minimumSpacing\":25,\"sides\":[{\"content\":{\"connectorIds\":[\"In1\"]},\"type\":\"ConnectorPlacement.EquallySpacedRectSide\",\"uuid\":\"d45e420a-c48a-4f64-96ce-c5c35bb4ca1a\"},{\"content\":{\"connectorIds\":[\"Out1\",\"Out2\"],\"side\":\"RIGHT\"},\"type\":\"ConnectorPlacement.EquallySpacedRectSide\",\"uuid\":\"a4e2bce0-d957-4e8d-907b-26e945724fec\"},{\"content\":{\"side\":\"TOP\"},\"type\":\"ConnectorPlacement.EquallySpacedRectSide\",\"uuid\":\"f887741f-84ea-4dc9-b916-61633ba77119\"},{\"content\":{\"connectorIds\":[\"Out3\"],\"side\":\"BOTTOM\"},\"type\":\"ConnectorPlacement.EquallySpacedRectSide\",\"uuid\":\"7b6530e5-14c5-4e05-baa0-f0dfe0680bf2\"}]},\"type\":\"ConnectorPlacement.EquallySpacedConnector\",\"uuid\":\"ffda6ec7-3a8c-4734-85c7-d4d2baf408ab\"}],\"packageUris\":[\"http://schema.mathworks.com/mf0/Connector/R2020b\"],\"version\":\"1.0\"}"
  Bus Element Out3 : Outport  PortName=ASP Effects Power
  Bus Element Out2 : Outport  Port=2  PortName=DSP Core Power
  Bus Element Out1 : Outport  Port=3  PortName=MCU Power
  wires:
  Bus Element In1/1 -> 9V 2.1mm Jack/1(9V DC)
  9V 2.1mm Jack/1(DC In) -> Power Bus/1(DC In)
  Power Bus/3(MCU Power) -> Bus Element Out1/1
  Power Bus/1(DSP Core Power) -> Bus Element Out2/1
  Power Bus/2(ASP Effects Power) -> Bus Element Out3/1

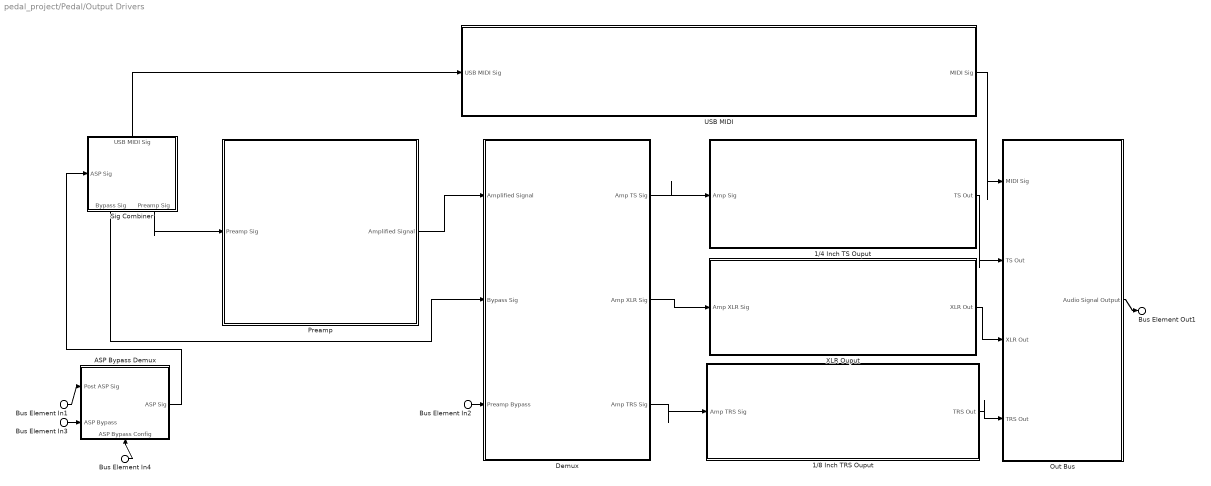
== system pedal_project/Pedal/Output Drivers ==
  Bus Element In1 : Inport  PortName=Post ASP Sig
  Bus Element In2 : Inport  Port=2  PortName=Preamp Bypass
  Bus Element In3 : Inport  Port=3  PortName=ASP Bypass
  Bus Element In4 : Inport  Port=4  PortName=ASP Bypass Config
  1/4 Inch TS Ouput : Subsystem
      settings: PortSchema="{\"entries\":[{\"content\":{\"headerSize\":26,\"margin\":15,\"minimumSpacing\":25,\"sides\":[{\"content\":{\"connectorIds\":[\"In1\"]},\"type\":\"ConnectorPlacement.EquallySpacedRectSide\",\"uuid\":\"d45e420a-c48a-4f64-96ce-c5c35bb4ca1a\"},{\"content\":{\"connectorIds\":[\"Out1\"],\"side\":\"RIGHT\"},\"type\":\"ConnectorPlacement.EquallySpacedRectSide\",\"uuid\":\"a4e2bce0-d957-4e8d-907b-26e945724fec\"},{\"content\":{\"side\":\"TOP\"},\"type\":\"ConnectorPlacement.EquallySpacedRectSide\",\"uuid\":\"f887741f-84ea-4dc9-b916-61633ba77119\"}]},\"type\":\"ConnectorPlacement.EquallySpacedConnector\",\"uuid\":\"ffda6ec7-3a8c-4734-85c7-d4d2baf408ab\"}],\"packageUris\":[\"http://schema.mathworks.com/mf0/Connector/R2020b\"],\"version\":\"1.0\"}"
  1/8 Inch TRS Ouput : Subsystem
      settings: PortSchema="{\"entries\":[{\"content\":{\"headerSize\":26,\"margin\":15,\"minimumSpacing\":25,\"sides\":[{\"content\":{\"connectorIds\":[\"In1\"]},\"type\":\"ConnectorPlacement.EquallySpacedRectSide\",\"uuid\":\"d45e420a-c48a-4f64-96ce-c5c35bb4ca1a\"},{\"content\":{\"connectorIds\":[\"Out1\"],\"side\":\"RIGHT\"},\"type\":\"ConnectorPlacement.EquallySpacedRectSide\",\"uuid\":\"a4e2bce0-d957-4e8d-907b-26e945724fec\"},{\"content\":{\"side\":\"TOP\"},\"type\":\"ConnectorPlacement.EquallySpacedRectSide\",\"uuid\":\"f887741f-84ea-4dc9-b916-61633ba77119\"}]},\"type\":\"ConnectorPlacement.EquallySpacedConnector\",\"uuid\":\"ffda6ec7-3a8c-4734-85c7-d4d2baf408ab\"}],\"packageUris\":[\"http://schema.mathworks.com/mf0/Connector/R2020b\"],\"version\":\"1.0\"}"
  ASP Bypass Demux : Subsystem
      settings: PortSchema="{\"entries\":[{\"content\":{\"headerSize\":26,\"margin\":15,\"minimumSpacing\":25,\"sides\":[{\"content\":{\"connectorIds\":[\"In2\",\"In3\"]},\"type\":\"ConnectorPlacement.EquallySpacedRectSide\",\"uuid\":\"d45e420a-c48a-4f64-96ce-c5c35bb4ca1a\"},{\"content\":{\"connectorIds\":[\"Out1\"],\"side\":\"RIGHT\"},\"type\":\"ConnectorPlacement.EquallySpacedRectSide\",\"uuid\":\"a4e2bce0-d957-4e8d-907b-26e945724fec\"},{\"content\":{\"side\":\"TOP\"},\"type\":\"ConnectorPlacement.EquallySpacedRectSide\",\"uuid\":\"f887741f-84ea-4dc9-b916-61633ba77119\"},{\"content\":{\"connectorIds\":[\"In1\"],\"side\":\"BOTTOM\"},\"type\":\"ConnectorPlacement.EquallySpacedRectSide\",\"uuid\":\"e9307776-dd5f-4e64-afa5-1474a492f2e5\"}]},\"type\":\"ConnectorPlacement.EquallySpacedConnector\",\"uuid\":\"ffda6ec7-3a8c-4734-85c7-d4d2baf408ab\"}],\"packageUris\":[\"http://schema.mathworks.com/mf0/Connector/R2020b\"],\"version\":\"1.0\"}"
  Demux : Subsystem
      settings: PortSchema="{\"entries\":[{\"content\":{\"headerSize\":26,\"margin\":15,\"minimumSpacing\":25,\"sides\":[{\"content\":{\"connectorIds\":[\"In1\",\"In2\",\"In3\"]},\"type\":\"ConnectorPlacement.EquallySpacedRectSide\",\"uuid\":\"d45e420a-c48a-4f64-96ce-c5c35bb4ca1a\"},{\"content\":{\"connectorIds\":[\"Out1\",\"Out2\",\"Out3\"],\"side\":\"RIGHT\"},\"type\":\"ConnectorPlacement.EquallySpacedRectSide\",\"uuid\":\"a4e2bce0-d957-4e8d-907b-26e945724fec\"},{\"content\":{\"side\":\"TOP\"},\"type\":\"ConnectorPlacement.EquallySpacedRectSide\",\"uuid\":\"f887741f-84ea-4dc9-b916-61633ba77119\"}]},\"type\":\"ConnectorPlacement.EquallySpacedConnector\",\"uuid\":\"ffda6ec7-3a8c-4734-85c7-d4d2baf408ab\"}],\"packageUris\":[\"http://schema.mathworks.com/mf0/Connector/R2020b\"],\"version\":\"1.0\"}"
  Out Bus : Subsystem
      settings: PortSchema="{\"entries\":[{\"content\":{\"headerSize\":26,\"margin\":15,\"minimumSpacing\":25,\"sides\":[{\"content\":{\"connectorIds\":[\"In1\",\"In2\",\"In3\",\"In4\"]},\"type\":\"ConnectorPlacement.EquallySpacedRectSide\",\"uuid\":\"d45e420a-c48a-4f64-96ce-c5c35bb4ca1a\"},{\"content\":{\"connectorIds\":[\"Out1\"],\"side\":\"RIGHT\"},\"type\":\"ConnectorPlacement.EquallySpacedRectSide\",\"uuid\":\"a4e2bce0-d957-4e8d-907b-26e945724fec\"},{\"content\":{\"side\":\"TOP\"},\"type\":\"ConnectorPlacement.EquallySpacedRectSide\",\"uuid\":\"f887741f-84ea-4dc9-b916-61633ba77119\"}]},\"type\":\"ConnectorPlacement.EquallySpacedConnector\",\"uuid\":\"ffda6ec7-3a8c-4734-85c7-d4d2baf408ab\"}],\"packageUris\":[\"http://schema.mathworks.com/mf0/Connector/R2020b\"],\"version\":\"1.0\"}"
  Preamp : Subsystem
      settings: PortSchema="{\"entries\":[{\"content\":{\"headerSize\":26,\"margin\":15,\"minimumSpacing\":25,\"sides\":[{\"content\":{\"connectorIds\":[\"In1\"]},\"type\":\"ConnectorPlacement.EquallySpacedRectSide\",\"uuid\":\"d45e420a-c48a-4f64-96ce-c5c35bb4ca1a\"},{\"content\":{\"connectorIds\":[\"Out1\"],\"side\":\"RIGHT\"},\"type\":\"ConnectorPlacement.EquallySpacedRectSide\",\"uuid\":\"a4e2bce0-d957-4e8d-907b-26e945724fec\"},{\"content\":{\"side\":\"TOP\"},\"type\":\"ConnectorPlacement.EquallySpacedRectSide\",\"uuid\":\"f887741f-84ea-4dc9-b916-61633ba77119\"}]},\"type\":\"ConnectorPlacement.EquallySpacedConnector\",\"uuid\":\"ffda6ec7-3a8c-4734-85c7-d4d2baf408ab\"}],\"packageUris\":[\"http://schema.mathworks.com/mf0/Connector/R2020b\"],\"version\":\"1.0\"}"
  Sig Combiner : Subsystem
      settings: PortSchema="{\"entries\":[{\"content\":{\"headerSize\":26,\"margin\":15,\"minimumSpacing\":25,\"sides\":[{\"content\":{\"connectorIds\":[\"In1\"]},\"type\":\"ConnectorPlacement.EquallySpacedRectSide\",\"uuid\":\"d45e420a-c48a-4f64-96ce-c5c35bb4ca1a\"},{\"content\":{\"side\":\"RIGHT\"},\"type\":\"ConnectorPlacement.EquallySpacedRectSide\",\"uuid\":\"a4e2bce0-d957-4e8d-907b-26e945724fec\"},{\"content\":{\"connectorIds\":[\"Out3\"],\"side\":\"TOP\"},\"type\":\"ConnectorPlacement.EquallySpacedRectSide\",\"uuid\":\"f887741f-84ea-4dc9-b916-61633ba77119\"},{\"content\":{\"connectorIds\":[\"Out1\",\"Out2\"],\"side\":\"BOTTOM\"},\"type\":\"ConnectorPlacement.EquallySpacedRectSide\",\"uuid\":\"570397c9-d201-4db7-92fc-733540865097\"}]},\"type\":\"ConnectorPlacement.EquallySpacedConnector\",\"uuid\":\"ffda6ec7-3a8c-4734-85c7-d4d2baf408ab\"}],\"packageUris\":[\"http://schema.mathworks.com/mf0/Connector/R2020b\"],\"version\":\"1.0\"}"
  USB MIDI : Subsystem
      settings: PortSchema="{\"entries\":[{\"content\":{\"headerSize\":26,\"margin\":15,\"minimumSpacing\":25,\"sides\":[{\"content\":{\"connectorIds\":[\"In1\"]},\"type\":\"ConnectorPlacement.EquallySpacedRectSide\",\"uuid\":\"d45e420a-c48a-4f64-96ce-c5c35bb4ca1a\"},{\"content\":{\"connectorIds\":[\"Out1\"],\"side\":\"RIGHT\"},\"type\":\"ConnectorPlacement.EquallySpacedRectSide\",\"uuid\":\"a4e2bce0-d957-4e8d-907b-26e945724fec\"},{\"content\":{\"side\":\"TOP\"},\"type\":\"ConnectorPlacement.EquallySpacedRectSide\",\"uuid\":\"f887741f-84ea-4dc9-b916-61633ba77119\"}]},\"type\":\"ConnectorPlacement.EquallySpacedConnector\",\"uuid\":\"ffda6ec7-3a8c-4734-85c7-d4d2baf408ab\"}],\"packageUris\":[\"http://schema.mathworks.com/mf0/Connector/R2020b\"],\"version\":\"1.0\"}"
  XLR Ouput : Subsystem
      settings: PortSchema="{\"entries\":[{\"content\":{\"headerSize\":26,\"margin\":15,\"minimumSpacing\":25,\"sides\":[{\"content\":{\"connectorIds\":[\"In1\"]},\"type\":\"ConnectorPlacement.EquallySpacedRectSide\",\"uuid\":\"d45e420a-c48a-4f64-96ce-c5c35bb4ca1a\"},{\"content\":{\"connectorIds\":[\"Out1\"],\"side\":\"RIGHT\"},\"type\":\"ConnectorPlacement.EquallySpacedRectSide\",\"uuid\":\"a4e2bce0-d957-4e8d-907b-26e945724fec\"},{\"content\":{\"side\":\"TOP\"},\"type\":\"ConnectorPlacement.EquallySpacedRectSide\",\"uuid\":\"f887741f-84ea-4dc9-b916-61633ba77119\"}]},\"type\":\"ConnectorPlacement.EquallySpacedConnector\",\"uuid\":\"ffda6ec7-3a8c-4734-85c7-d4d2baf408ab\"}],\"packageUris\":[\"http://schema.mathworks.com/mf0/Connector/R2020b\"],\"version\":\"1.0\"}"
  Bus Element Out1 : Outport  PortName=Audio Signal Output
  wires:
  Preamp/1(Amplified Signal) -> Demux/1(Amplified Signal)
  Out Bus/1(Audio Signal Output) -> Bus Element Out1/1
  1/4 Inch TS Ouput/1(TS Out) -> Out Bus/2(TS Out)
  XLR Ouput/1(XLR Out) -> Out Bus/3(XLR Out)
  1/8 Inch TRS Ouput/1(TRS Out) -> Out Bus/4(TRS Out)
  Bus Element In2/1 -> Demux/3(Preamp Bypass)
  Demux/1(Amp TS Sig) -> 1/4 Inch TS Ouput/1(Amp Sig)
  Demux/2(Amp XLR Sig) -> XLR Ouput/1(Amp XLR Sig)
  Demux/3(Amp TRS Sig) -> 1/8 Inch TRS Ouput/1(Amp TRS Sig)
  Sig Combiner/3(USB MIDI Sig) -> USB MIDI/1(USB MIDI Sig)
  Sig Combiner/2(Preamp Sig) -> Preamp/1(Preamp Sig)
  Sig Combiner/1(Bypass Sig) -> Demux/2(Bypass Sig)
  USB MIDI/1(MIDI Sig) -> Out Bus/1(MIDI Sig)
  Bus Element In3/1 -> ASP Bypass Demux/3(ASP Bypass)
  Bus Element In1/1 -> ASP Bypass Demux/2(Post ASP Sig)
  ASP Bypass Demux/1(ASP Sig) -> Sig Combiner/1(ASP Sig)
  Bus Element In4/1 -> ASP Bypass Demux/1(ASP Bypass Config)

== system pedal_project/Phone/Software Application ==
  Configurable Analog Processing : Subsystem
      settings: PortSchema="{\"entries\":[{\"content\":{\"headerSize\":26,\"margin\":15,\"minimumSpacing\":25,\"sides\":[{\"content\":{},\"type\":\"ConnectorPlacement.EquallySpacedRectSide\",\"uuid\":\"d45e420a-c48a-4f64-96ce-c5c35bb4ca1a\"},{\"content\":{\"connectorIds\":[\"Out1\"],\"side\":\"RIGHT\"},\"type\":\"ConnectorPlacement.EquallySpacedRectSide\",\"uuid\":\"a4e2bce0-d957-4e8d-907b-26e945724fec\"},{\"content\":{\"side\":\"TOP\"},\"type\":\"ConnectorPlacement.EquallySpacedRectSide\",\"uuid\":\"f887741f-84ea-4dc9-b916-61633ba77119\"}]},\"type\":\"ConnectorPlacement.EquallySpacedConnector\",\"uuid\":\"ffda6ec7-3a8c-4734-85c7-d4d2baf408ab\"}],\"packageUris\":[\"http://schema.mathworks.com/mf0/Connector/R2020b\"],\"version\":\"1.0\"}"
  Configurable Digital Processing : Subsystem
      settings: PortSchema="{\"entries\":[{\"content\":{\"headerSize\":26,\"margin\":15,\"minimumSpacing\":25,\"sides\":[{\"content\":{\"connectorIds\":[\"Out1\"]},\"type\":\"ConnectorPlacement.EquallySpacedRectSide\",\"uuid\":\"d45e420a-c48a-4f64-96ce-c5c35bb4ca1a\"},{\"content\":{\"side\":\"RIGHT\"},\"type\":\"ConnectorPlacement.EquallySpacedRectSide\",\"uuid\":\"a4e2bce0-d957-4e8d-907b-26e945724fec\"},{\"content\":{\"side\":\"TOP\"},\"type\":\"ConnectorPlacement.EquallySpacedRectSide\",\"uuid\":\"f887741f-84ea-4dc9-b916-61633ba77119\"}]},\"type\":\"ConnectorPlacement.EquallySpacedConnector\",\"uuid\":\"ffda6ec7-3a8c-4734-85c7-d4d2baf408ab\"}],\"packageUris\":[\"http://schema.mathworks.com/mf0/Connector/R2020b\"],\"version\":\"1.0\"}"
  Effects Validation and Upload : Subsystem
      settings: PortSchema="{\"entries\":[{\"content\":{\"headerSize\":26,\"margin\":15,\"minimumSpacing\":25,\"sides\":[{\"content\":{\"connectorIds\":[\"In1\",\"In2\"]},\"type\":\"ConnectorPlacement.EquallySpacedRectSide\",\"uuid\":\"d45e420a-c48a-4f64-96ce-c5c35bb4ca1a\"},{\"content\":{\"connectorIds\":[\"Out1\"],\"side\":\"RIGHT\"},\"type\":\"ConnectorPlacement.EquallySpacedRectSide\",\"uuid\":\"a4e2bce0-d957-4e8d-907b-26e945724fec\"},{\"content\":{\"side\":\"TOP\"},\"type\":\"ConnectorPlacement.EquallySpacedRectSide\",\"uuid\":\"f887741f-84ea-4dc9-b916-61633ba77119\"}]},\"type\":\"ConnectorPlacement.EquallySpacedConnector\",\"uuid\":\"ffda6ec7-3a8c-4734-85c7-d4d2baf408ab\"}],\"packageUris\":[\"http://schema.mathworks.com/mf0/Connector/R2020b\"],\"version\":\"1.0\"}"
  Bus Element Out1 : Outport  PortName=Configuration Upload Packets
  wires:
  Effects Validation and Upload/1(Configuration Upload Packets) -> Bus Element Out1/1
  Configurable Analog Processing/1(Analog Effects Configuration) -> Effects Validation and Upload/1(Analog Effects Configuration)
  Configurable Digital Processing/1(Digital Effects Configuration) -> Effects Validation and Upload/2(Digital Effects Configuration)

== system pedal_project/Phone/USB Output Driver ==
  Bus Element In1 : Inport  PortName=Configuration Upload Packets
  Bus Element Out1 : Outport  PortName=App Control Packets

== system pedal_project/Wall Power/120V Wall Output ==
  Bus Element Out1 : Outport  PortName=Wall Power

== system pedal_project/Wall Power/9V DC Power Supply ==
  Bus Element In1 : Inport  PortName=Wall Power
  Bus Element Out1 : Outport  PortName=9V DC

== system pedal_project/Pedal/Analog Front End/1//4 Inch TS Input Jack ==
  Bus Element In1 : Inport  PortName=Instrument Signal
  Bus Element Out1 : Outport  PortName=Input Signal
